simulink model "ConverterWithPID"  (R2023a)
settings: Solver=ode23tb  StartTime=0.0  StopTime=0.1  FixedStep=0.0000001  MaxStep=0.0000001  RelTol=1e-4  AbsTol=1e-4
values from neighbouring files (symbols this model uses):
  C = [0 1]    [BoostConverterHybrid.m]    (also in boost_converter_sfcnv3.m = u(4); params_dcdc.m = 0.0001; params_forEVcharge.m = 0.00010675)
  D = u(2)    [boost_converter_sfcnv3.m]    (also in params_dcdc.m = 0.5; params_forEVcharge.m = 0.625)
  E = u(1)    [boost_converter_sfcnv3.m]    (also in params_dcdc.m = 20; params_forEVcharge.m = 90)
  L = 1    [BoostConverterHybrid.m]    (also in boost_converter_sfcnv3.m = u(3); params_dcdc.m = 3e-05; params_forEVcharge.m = 0.008945)
  R = 1    [BoostConverterHybrid.m]    (also in boost_converter_sfcnv3.m = u(5); params_dcdc.m = 10; params_forEVcharge.m = 48.48)
  T = 298    [parameterEstimationv2.m]    (also in params_dcdc.m = 5e-05; params_forEVcharge.m = 1e-05)
undefined symbols (not defined in the file or in its folder): Vs
libraries: slpidlib x2, spsPWMGeneratorDCDCLib x2, simulink x1
settings Model: Creator=lucea  LastModifiedBy=gabrielcrisan

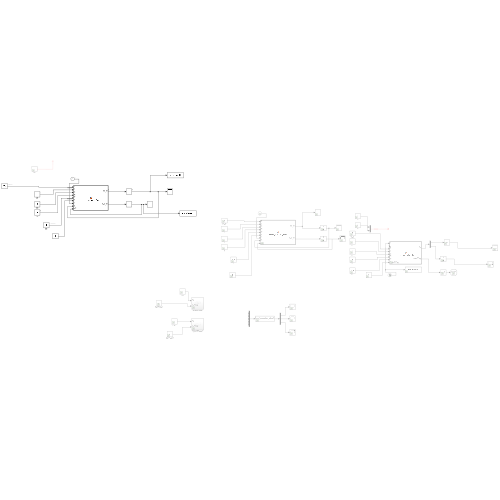
[thumbnail: Simulink's stored preview of the top-level diagram]
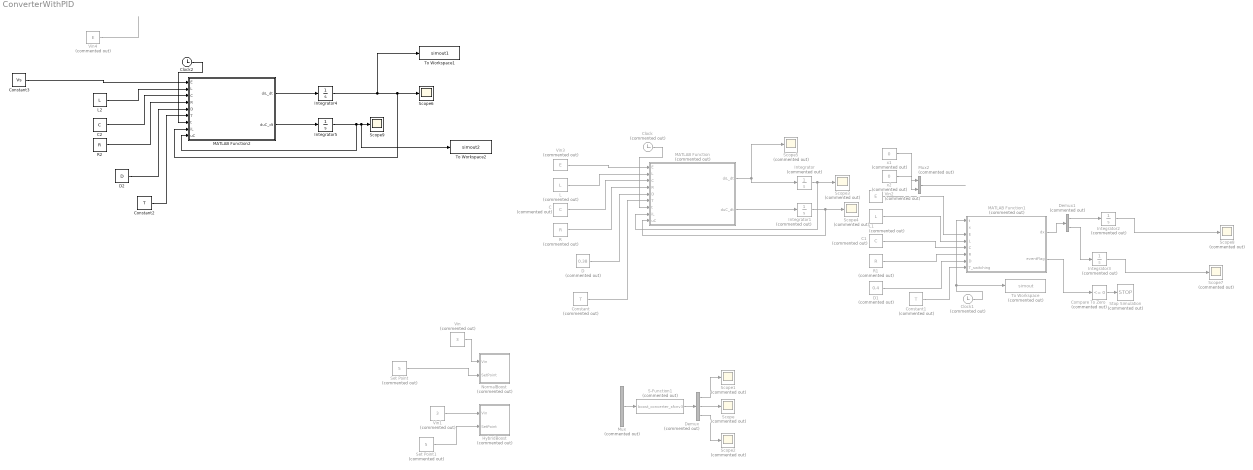
== system ConverterWithPID ==
  C : Constant  Commented=on  Value=C
  C1 : Constant  Commented=on  Value=C
  C2 : Constant  Value=C
  Clock : Clock  Commented=on
  Clock1 : Clock  Commented=on
  Clock2 : Clock
  Compare To Zero : simulink/Logic and Bit Operations/Compare To Zero  Commented=on  relop=<=  OutDataTypeStr=boolean
  Constant : Constant  Commented=on  Value=T
  Constant1 : Constant  Commented=on  Value=T
  Constant2 : Constant  Value=T
  Constant3 : Constant  Value=Vs
  D : Constant  Commented=on  Value=0.38
  D1 : Constant  Commented=on  Value=0.4
  D2 : Constant  Value=D
  Demux : Demux  Commented=on  Outputs=3
  Demux1 : Demux  Commented=on  Outputs=2
  HybridBoost : Subsystem  Commented=on
  Integrator{,1..3} (4 alike) : Integrator  Commented=on
  Integrator4 : Integrator
  Integrator5 : Integrator
  L : Constant  Commented=on  Value=L
  L1 : Constant  Commented=on  Value=L
  L2 : Constant  Value=L
  MATLAB Function : MATLAB Function  Commented=on  TreatAsAtomicUnit=on
  MATLAB Function1 : MATLAB Function  Commented=on  TreatAsAtomicUnit=on
  MATLAB Function2 : MATLAB Function  TreatAsAtomicUnit=on
  Mux : Mux  Commented=on  Inputs=5
  Mux2 : Mux  Commented=on  Inputs=2
  NormalBoost : Subsystem  Commented=on
  R : Constant  Commented=on  Value=R
  R1 : Constant  Commented=on  Value=R
  R2 : Constant  Value=R
  S-Function1 : S-Function  Commented=on  FunctionName=boost_converter_sfcnv3  SFunctionDeploymentMode=off  EnableBusSupport=off
  Scope{,1..5,7..8} (8 alike) : Scope  Commented=on
  Scope6 : Scope
  Scope9 : Scope
  Set Point : Constant  Commented=on  Value=5
  Set Point1 : Constant  Commented=on  Value=5
  Stop Simulation : Stop  Commented=on
  To Workspace : ToWorkspace  Commented=on  VariableName=simout  SaveFormat=Timeseries  SampleTime=-1
  To Workspace1 : ToWorkspace  VariableName=simout1  SaveFormat=Timeseries  SampleTime=-1
  To Workspace2 : ToWorkspace  VariableName=simout2  SaveFormat=Timeseries  SampleTime=-1
  Vin : Constant  Commented=on  Value=3
  Vin1 : Constant  Commented=on  Value=3
  Vin2 : Constant  Commented=on  Value=E
  Vin3 : Constant  Commented=on  Value=E
  Vin4 : Constant  Commented=on  Value=E
  x1 : Constant  Commented=on  Value=0
  x2 : Constant  Commented=on  Value=0
  wires:
  Vin/1 -> NormalBoost/1(Vin)
  Set Point/1 -> NormalBoost/2(SetPoint)
  Vin1/1 -> HybridBoost/1(Vin)
  Set Point1/1 -> HybridBoost/2(SetPoint)
  Mux/1 -> S-Function1/1
  S-Function1/1 -> Demux/1
  Demux/1 -> Scope1/1
  Demux/3 -> Scope2/1
  Demux/2 -> Scope/1
  L/1 -> MATLAB Function/2(L)
  C/1 -> MATLAB Function/3(C)
  D/1 -> MATLAB Function/5(D)
  R/1 -> MATLAB Function/4(R)
  Vin3/1 -> MATLAB Function/1(E)
  MATLAB Function/1(diL_dt) -> Integrator/1, Scope5/1
  MATLAB Function/2(duC_dt) -> Integrator1/1
  Integrator/1 -> MATLAB Function/8(iL), Scope3/1
  Integrator1/1 -> MATLAB Function/9(uC), Scope4/1
  Clock/1 -> MATLAB Function/7(t)
  Constant/1 -> MATLAB Function/6(T)
  Constant1/1 -> MATLAB Function1/8(T_switching)
  Mux2/1 -> ?
  x1/1 -> Mux2/1
  x2/1 -> Mux2/2
  Clock1/1 -> To Workspace/1, MATLAB Function1/1(t)
  Integrator2/1 -> Scope8/1
  Vin2/1 -> MATLAB Function1/3(E)
  R1/1 -> MATLAB Function1/6(R)
  D1/1 -> MATLAB Function1/7(D)
  C1/1 -> MATLAB Function1/5(C)
  L1/1 -> MATLAB Function1/4(L)
  MATLAB Function1/1(dx) -> Demux1/1
  Demux1/1 -> Integrator2/1
  Integrator3/1 -> Scope7/1
  Demux1/2 -> Integrator3/1
  MATLAB Function1/2(eventFlag) -> Compare To Zero/1
  Compare To Zero/1 -> Stop Simulation/1
  L2/1 -> MATLAB Function2/2(L)
  R2/1 -> MATLAB Function2/4(R)
  D2/1 -> MATLAB Function2/5(D)
  C2/1 -> MATLAB Function2/3(C)
  Vin4/1 -> ?
  Constant2/1 -> MATLAB Function2/6(T)
  MATLAB Function2/1(diL_dt) -> Integrator4/1
  Clock2/1 -> MATLAB Function2/7(t)
  Integrator5/1 -> To Workspace2/1, Scope9/1, MATLAB Function2/9(uC)
  Integrator4/1 -> To Workspace1/1, Scope6/1, MATLAB Function2/8(iL)
  MATLAB Function2/2(duC_dt) -> Integrator5/1
  Constant3/1 -> MATLAB Function2/1(E)

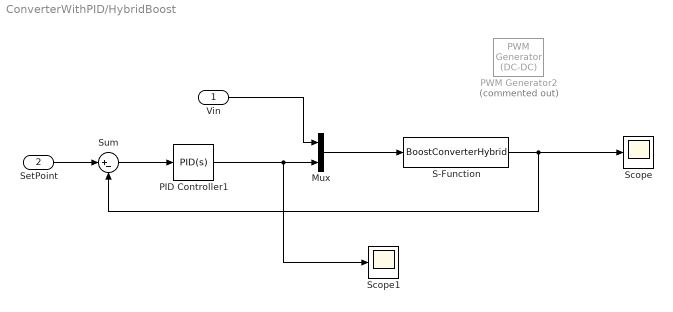
== system ConverterWithPID/HybridBoost ==
  Vin : Inport
  SetPoint : Inport  Port=2
  Mux : Mux  Inputs=2
  PID Controller1 : slpidlib/PID Controller  Controller=PID  Form=Parallel  TimeDomain=Continuous-time  UseExternalTs=off  SampleTime=-1  IntegratorMethod=Forward Euler  FilterMethod=Forward Euler  ControllerParametersSource=internal  P=10  I=0.2  UseKiTs=off  D=0  N=100  UseFilter=on  TunerSelectOption=Transfer Function Based (PID Tuner App)  InitialConditionSource=internal  InitialConditionForIntegrator=0  InitialConditionForFilter=0  DifferentiatorICPrevScaledInput=0  ExternalReset=none  TrackingMode=off  Kt=1  LimitOutput=off  SatLimitsSource=internal  UpperSaturationLimit=inf  LowerSaturationLimit=-inf  LinearizeAsGain=on  AntiWindupMode=none  Kb=1  LimitIntegrator=off  UpperIntegratorSaturationLimit=inf  LowerIntegratorSaturationLimit=-inf  POutMin=[]  POutMax=[]  IOutMin=[]  IOutMax=[]  DOutMin=[]  DOutMax=[]  NOutMin=[]  NOutMax=[]  SumOutMin=[]  SumOutMax=[]  SaturationOutMin=[]  SaturationOutMax=[]  PParamMin=[]  PParamMax=[]  IParamMin=[]  IParamMax=[]  DParamMin=[]  DParamMax=[]  NParamMin=[]  NParamMax=[]  KbParamMin=[]  KbParamMax=[]  KtParamMin=[]  KtParamMax=[]  KbOutMin=[]  KbOutMax=[]  KtOutMin=[]  KtOutMax=[]  IntegratorOutMin=[]  IntegratorOutMax=[]  FilterOutMin=[]  FilterOutMax=[]  SumI1OutMin=[]  SumI1OutMax=[]  SumI2OutMin=[]  SumI2OutMax=[]  SumI3OutMin=[]  SumI3OutMax=[]  SumI4OutMin=[]  SumI4OutMax=[]  SumDOutMin=[]  SumDOutMax=[]  DifferentiatorOutMin=[]  DifferentiatorOutMax=[]  FilterDiffOutCoefMin=[]  FilterDiffOutCoefMax=[]  ReciprocalOutMin=[]  ReciprocalOutMax=[]  SumDenOutMin=[]  SumDenOutMax=[]  SumNumOutMin=[]  SumNumOutMax=[]  DivideOutMin=[]  DivideOutMax=[]  UdiffTsProdOutMin=[]  UdiffTsProdOutMax=[]  NTsProdOutMin=[]  NTsProdOutMax=[]  UintegralTsProdOutMin=[]  UintegralTsProdOutMax=[]  UngainTsProdOutMin=[]  UngainTsProdOutMax=[]  ClampingZeroOutDataTypeStr=Inherit: Inherit via back propagation  ClampingZeroOutMin=[]  ClampingZeroOutMax=[]  FilterDenConstantOutDataTypeStr=Inherit: Inherit via back propagation  FilterDenConstantOutMin=[]  FilterDenConstantOutMax=[]  PCopyOutDataTypeStr=Inherit: Inherit via back propagation  PCopyOutMin=[]  PCopyOutMax=[]  NCopyOutDataTypeStr=Inherit: Inherit via back propagation  NCopyOutMin=[]  NCopyOutMax=[]  IntegratorContinuousStateAttributes=''  IntegratorStateMustResolveToSignalObject=off  IntegratorRTWStateStorageClass=Auto  FilterContinuousStateAttributes=''  FilterStateMustResolveToSignalObject=off  FilterRTWStateStorageClass=Auto  ParallelPVariant=InternalParameters  IdealPVariant=Disabled  IVariant=InternalParameters  DVariant=InternalParameters  IntegratorVariant=Continuous  SatVariant=Disabled  AWVariant=Passthrough  PCopyVariant=Disabled  TRVariant=Disabled  FdbkBlocksVariant=Forward  IdealPFdbkVariant=Disabled  SatFdbkVariant=Disabled  DerivativeFilterVariant=ContFilter  NVariant=InternalParameters  NCopyVariant=Disabled  FilterICVariant=InternalICsFilter  IntegratorICVariant=InternalICs  ExternalResetVariant=Disabled  TRSumVariant=Passthrough  SumFdbkVariant=Disabled  SumVariant=Sum_PID  TsampFilterVariant=InternalTs  TsampNgainVariant=Passthrough  TsampIntegralVariant=Disabled_SignalSpec  ExternalSaturationOutDataTypeStr=Inherit: Same as second input
  PWM Generator2 : spsPWMGeneratorDCDCLib/PWM Generator (DC-DC)  Commented=on  Fsw=100  Ts=0
  S-Function : S-Function  FunctionName=BoostConverterHybrid  SFunctionDeploymentMode=off  EnableBusSupport=off
  Scope : Scope
  Scope1 : Scope
  Sum : Sum  Inputs=|+-
  wires:
  SetPoint/1 -> Sum/1
  S-Function/1 -> Scope/1, Sum/2
  Vin/1 -> Mux/1
  Sum/1 -> PID Controller1/1
  Mux/1 -> S-Function/1
  PID Controller1/1 -> Mux/2, Scope1/1

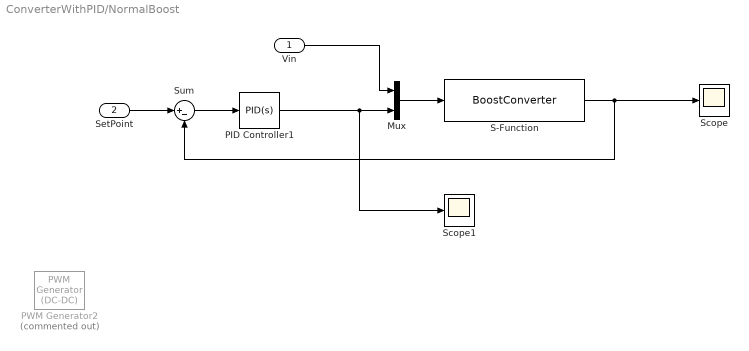
== system ConverterWithPID/NormalBoost ==
  Vin : Inport
  SetPoint : Inport  Port=2
  Mux : Mux  Inputs=2
  PID Controller1 : slpidlib/PID Controller  Controller=PID  Form=Parallel  TimeDomain=Continuous-time  UseExternalTs=off  SampleTime=-1  IntegratorMethod=Forward Euler  FilterMethod=Forward Euler  ControllerParametersSource=internal  P=10  I=0.2  UseKiTs=off  D=0  N=100  UseFilter=on  TunerSelectOption=Transfer Function Based (PID Tuner App)  InitialConditionSource=internal  InitialConditionForIntegrator=0  InitialConditionForFilter=0  DifferentiatorICPrevScaledInput=0  ExternalReset=none  TrackingMode=off  Kt=1  LimitOutput=off  SatLimitsSource=internal  UpperSaturationLimit=inf  LowerSaturationLimit=-inf  LinearizeAsGain=on  AntiWindupMode=none  Kb=1  LimitIntegrator=off  UpperIntegratorSaturationLimit=inf  LowerIntegratorSaturationLimit=-inf  POutMin=[]  POutMax=[]  IOutMin=[]  IOutMax=[]  DOutMin=[]  DOutMax=[]  NOutMin=[]  NOutMax=[]  SumOutMin=[]  SumOutMax=[]  SaturationOutMin=[]  SaturationOutMax=[]  PParamMin=[]  PParamMax=[]  IParamMin=[]  IParamMax=[]  DParamMin=[]  DParamMax=[]  NParamMin=[]  NParamMax=[]  KbParamMin=[]  KbParamMax=[]  KtParamMin=[]  KtParamMax=[]  KbOutMin=[]  KbOutMax=[]  KtOutMin=[]  KtOutMax=[]  IntegratorOutMin=[]  IntegratorOutMax=[]  FilterOutMin=[]  FilterOutMax=[]  SumI1OutMin=[]  SumI1OutMax=[]  SumI2OutMin=[]  SumI2OutMax=[]  SumI3OutMin=[]  SumI3OutMax=[]  SumI4OutMin=[]  SumI4OutMax=[]  SumDOutMin=[]  SumDOutMax=[]  DifferentiatorOutMin=[]  DifferentiatorOutMax=[]  FilterDiffOutCoefMin=[]  FilterDiffOutCoefMax=[]  ReciprocalOutMin=[]  ReciprocalOutMax=[]  SumDenOutMin=[]  SumDenOutMax=[]  SumNumOutMin=[]  SumNumOutMax=[]  DivideOutMin=[]  DivideOutMax=[]  UdiffTsProdOutMin=[]  UdiffTsProdOutMax=[]  NTsProdOutMin=[]  NTsProdOutMax=[]  UintegralTsProdOutMin=[]  UintegralTsProdOutMax=[]  UngainTsProdOutMin=[]  UngainTsProdOutMax=[]  ClampingZeroOutDataTypeStr=Inherit: Inherit via back propagation  ClampingZeroOutMin=[]  ClampingZeroOutMax=[]  FilterDenConstantOutDataTypeStr=Inherit: Inherit via back propagation  FilterDenConstantOutMin=[]  FilterDenConstantOutMax=[]  PCopyOutDataTypeStr=Inherit: Inherit via back propagation  PCopyOutMin=[]  PCopyOutMax=[]  NCopyOutDataTypeStr=Inherit: Inherit via back propagation  NCopyOutMin=[]  NCopyOutMax=[]  IntegratorContinuousStateAttributes=''  IntegratorStateMustResolveToSignalObject=off  IntegratorRTWStateStorageClass=Auto  FilterContinuousStateAttributes=''  FilterStateMustResolveToSignalObject=off  FilterRTWStateStorageClass=Auto  ParallelPVariant=InternalParameters  IdealPVariant=Disabled  IVariant=InternalParameters  DVariant=InternalParameters  IntegratorVariant=Continuous  SatVariant=Disabled  AWVariant=Passthrough  PCopyVariant=Disabled  TRVariant=Disabled  FdbkBlocksVariant=Forward  IdealPFdbkVariant=Disabled  SatFdbkVariant=Disabled  DerivativeFilterVariant=ContFilter  NVariant=InternalParameters  NCopyVariant=Disabled  FilterICVariant=InternalICsFilter  IntegratorICVariant=InternalICs  ExternalResetVariant=Disabled  TRSumVariant=Passthrough  SumFdbkVariant=Disabled  SumVariant=Sum_PID  TsampFilterVariant=InternalTs  TsampNgainVariant=Passthrough  TsampIntegralVariant=Disabled_SignalSpec  ExternalSaturationOutDataTypeStr=Inherit: Same as second input
  PWM Generator2 : spsPWMGeneratorDCDCLib/PWM Generator (DC-DC)  Commented=on  Fsw=100  Ts=0
  S-Function : S-Function  FunctionName=BoostConverter  SFunctionDeploymentMode=off  EnableBusSupport=off
  Scope : Scope
  Scope1 : Scope
  Sum : Sum  Inputs=|+-
  wires:
  Mux/1 -> S-Function/1
  Sum/1 -> PID Controller1/1
  Vin/1 -> Mux/1
  S-Function/1 -> Sum/2, Scope/1
  SetPoint/1 -> Sum/1
  PID Controller1/1 -> Scope1/1, Mux/2

== matlab function ConverterWithPID/MATLAB Function1 ==
  data: t input; x input; dx output; E input; L input; C input; R input; D input; T_switching input; eventFlag output
function [dx, eventFlag] = boost_converter_slx(t, x, E, L, C, R, D, T_switching)
    % States
    iL = x(1);  
    uC = x(2);  

    % Calculate current interval
    t_mod = mod(t, T_switching);
    if t_mod < D * T_switching
        interval = 1;  % Switch is on
    else
        interval = 2;  % Switch is off
    end

    % Calculate derivatives based on interval
    if interval == 1
        diL_dt = E / L;
        duC_dt = -uC / (R * C);
    elseif interval == 2
        diL_dt = (E - uC) / L;
        duC_dt = (iL - uC / R) / C;
    else
        % Additional interval logic if needed
        diL_dt = 0;
        duC_dt = 0;
    end

    % Check event condition (iL reaching zero)
    eventFlag = iL <= 0;

    % Output derivatives and event flag
    dx = [diL_dt; duC_dt];
end

== matlab function ConverterWithPID/MATLAB Function ==
  settings: updateMethod=DISCRETE
  data: E input; L input; C input; R input; D input; T input; t input; diL_dt output; iL input; uC input; duC_dt output
function [diL_dt, duC_dt] = boost_converter_func(E, L, C, R, D, T, t, iL, uC)
    
    persistent t_last_switch interval

    if isempty(t_last_switch)
        t_last_switch = 0;
        interval = 1;  % Start with switch on
    end

    t_since_switch = t - t_last_switch;

    if interval == 1 && t_since_switch >= D * T
        interval = 2;  % Switch off
        t_last_switch = t;
    elseif interval == 2 && t_since_switch >= (1 - D) * T
        interval = 1;  % Switch on
        t_last_switch = t;
    end

    if interval == 1
        % Switch is on
        diL_dt = (E - uC) / L;
        duC_dt = iL / C;
    else
        % Switch is off
        diL_dt = -uC / L;
        duC_dt = (iL - uC / R) / C;
    end
end

== matlab function ConverterWithPID/MATLAB Function2 ==
  settings: updateMethod=DISCRETE
  data: E input; L input; C input; R input; D input; T input; t input; diL_dt output; iL input; uC input; duC_dt output
function [diL_dt, duC_dt] = boost_converter_func(E, L, C, R, D, T, t, iL, uC)
    
    persistent t_last_switch interval

    if isempty(t_last_switch)
        t_last_switch = 0;
        interval = 1;  % Start with switch on
    end

    t_since_switch = t - t_last_switch;

    if interval == 1 && t_since_switch >= D * T
        interval = 2;  % Switch off
        t_last_switch = t;
    elseif interval == 2 && t_since_switch >= (1 - D) * T
        interval = 3;  % Enter discontinuous mode (if applicable)
        t_last_switch = t;
    elseif interval == 3 && t_since_switch >= (1 - D) * T
        interval = 1;  % Switch on again
        t_last_switch = t;
    end

    % Initialize outputs
    diL_dt = 0;
    duC_dt = 0;

    switch interval
        case 1  % Switch is on, Diode is off
            diL_dt = E / L;
            duC_dt = -uC / (R * C);
        case 2  % Switch is off, Diode is on
            diL_dt = (E - uC) / L;
            duC_dt = (iL - uC / R) / C;
        case 3  % Discontinuous mode, both switch and diode off
            diL_dt = 0;
            duC_dt = -uC / (R * C);
    end
end
